simulink model "set_point_DISCRETO2"  (R2023b)
settings: Solver=VariableStepAuto  StartTime=0.0  StopTime=10.0  RelTol=1e-3
values from neighbouring files (symbols this model uses):
  r = 120    [constantes.m]
  Ts = 2*pi/(10*5000)    (= 0.000125663706144)    [constantes.m]    (also in test_polos_PID.m = 40)
undefined symbols (not defined in the file or in its folder): DiscIntNeverNeededParam
settings Model: Creator=Nahuel  LastModifiedBy=Nahuel

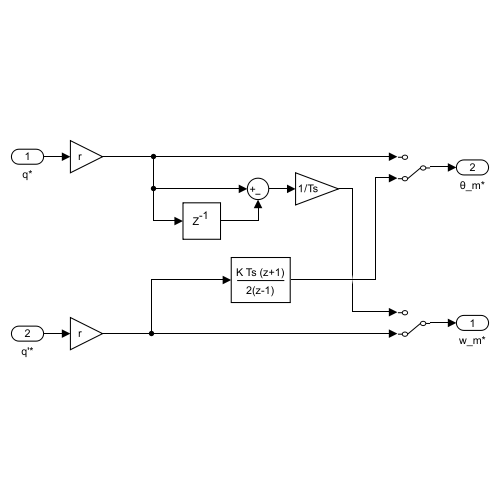
[thumbnail: Simulink's stored preview of the top-level diagram]
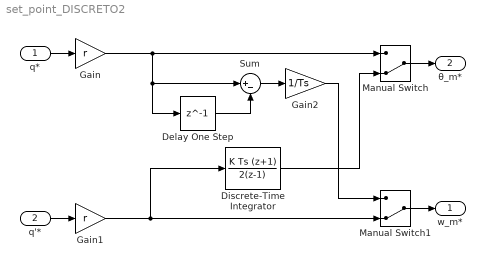
== system set_point_DISCRETO2 ==
  q* : Inport
  q'* : Inport  Port=2
  Delay One Step : Delay  DelayLength=1
  Discrete-Time Integrator : DiscreteIntegrator  IntegratorMethod=Integration: Trapezoidal  SampleTime=Ts  ICPrevOutput=DiscIntNeverNeededParam  ICPrevScaledInput=DiscIntNeverNeededParam
  Gain : Gain  Gain=r
  Gain1 : Gain  Gain=r
  Gain2 : Gain  Gain=1/Ts
  Manual Switch : ManualSwitch  CurrentSetting=0
  Manual Switch1 : ManualSwitch  CurrentSetting=0
  Sum : Sum  Inputs=|+-
  w_m* : Outport
  θ_m* : Outport  Port=2
  wires:
  Gain/1 -> Delay One Step/1, Sum/1, Manual Switch/1
  q'*/1 -> Gain1/1
  Sum/1 -> Gain2/1
  Manual Switch/1 -> θ_m*/1
  Discrete-Time Integrator/1 -> Manual Switch/2
  Gain1/1 -> Discrete-Time Integrator/1, Manual Switch1/2
  Manual Switch1/1 -> w_m*/1
  q*/1 -> Gain/1
  Delay One Step/1 -> Sum/2
  Gain2/1 -> Manual Switch1/1
